simulink subsystem "vecNorm"  (R2024b)
settings: Solver=VariableStepAuto  StartTime=0.0  StopTime=10.0  RelTol=1e-3
settings Model: Creator=ricca  LastModifiedBy=ricca

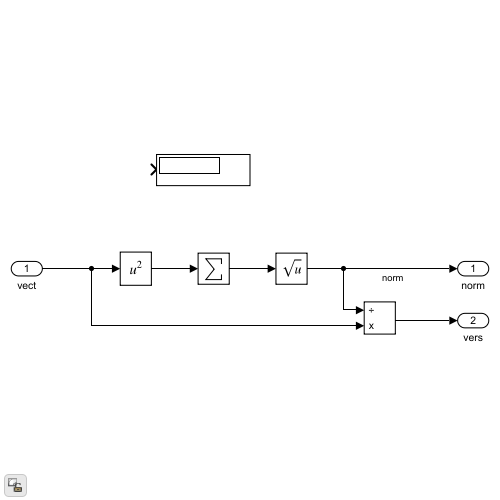
[thumbnail: Simulink's stored preview of the top-level diagram]
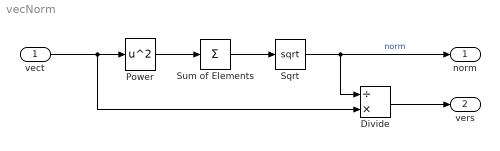
== system vecNorm ==
  vect : Inport
  Divide : Product  Inputs=/*
  Power : Math  Operator=square
  Sqrt : Sqrt
  Sum of Elements : Sum  Inputs=+
  norm : Outport
  vers : Outport  Port=2
  wires:
  Sum of Elements/1 -> Sqrt/1
  Power/1 -> Sum of Elements/1
  vect/1 -> Divide/2, Power/1
  Sqrt/1 -> Divide/1, norm/1  "norm"
  Divide/1 -> vers/1
